simulink library "mylib"  (Simulink 6.0)
settings: Solver=ode45  StartTime=0.0  StopTime=10.0  RelTol=1e-3
libraries: other_lib x2, simulink x1
settings Model: Creator=awarlock  LastModifiedBy=awarlock  ExtModeAutoUpdateStatusClock=off
settings DebuggingCC: CheckExecutionContextPreStartOutputMsg=on  CheckExecutionContextRuntimeOutputMsg=on
settings SFSimCC: SFSimApplyToAllLibs=on  SFSimBuildMode=Incremental

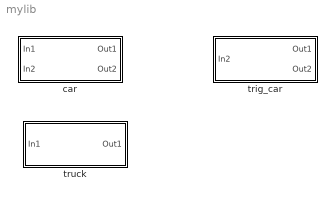
== system mylib ==
  car : Subsystem  TreatAsAtomicUnit=on  PropExecContextAcrossSSBoundary=on
  trig_car : Subsystem  TreatAsAtomicUnit=on  PropExecContextAcrossSSBoundary=on
  truck : Subsystem  TreatAsAtomicUnit=on  PropExecContextAcrossSSBoundary=on

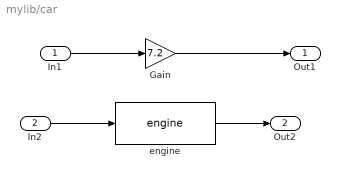
== system mylib/car ==
  In1 : Inport  LatchInput=off
  In2 : Inport  Port=2  LatchInput=off
  Gain : Gain  Gain=7.2
  engine : other_lib/engine
  Out1 : Outport
  Out2 : Outport  Port=2
  wires:
  In1/1 -> Gain/1
  In2/1 -> engine/1
  engine/1 -> Out2/1
  Gain/1 -> Out1/1

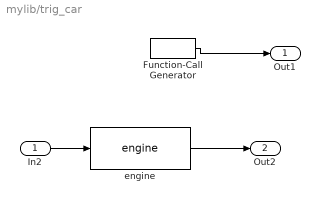
== system mylib/trig_car ==
  In2 : Inport  LatchInput=off
  Function-Call Generator : simulink/Ports & Subsystems/Function-Call Generator  sample_time=1  numberOfIterations=1
  engine : other_lib/engine
  Out1 : Outport
  Out2 : Outport  Port=2
  wires:
  engine/1 -> Out2/1
  In2/1 -> engine/1
  Function-Call Generator/1 -> Out1/1

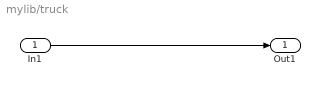
== system mylib/truck ==
  In1 : Inport  LatchInput=off
  Out1 : Outport
  wires:
  In1/1 -> Out1/1
